simulink model "scars_model."  (R2019b)
settings: Solver=FixedStepAuto  StartTime=0.0  StopTime=TFinal  FixedStep=dT  MaxStep=1  MinStep=dT  RelTol=1e-3
model workspace (MAT data in the model file):
  actuators = 0
values from neighbouring files (symbols this model uses):
  decsec = decyear(2000,1,1,12,0,1) - decyear(2000,1,1,12,0,0)    [SCARSSetup.m]    (also in pwsat2_setup.m; pwsat2_tle.m; scars_setup.m)
  decstart = decyear(utc)    [SCARSSetup.m]    (also in pwsat2_setup.m; pwsat2_tle.m; scars_setup.m)
  forcesBody = [0 0 0]    [SCARSSetup.m]    (also in pwsat2_setup.m; scars_setup.m)
  initMoments = [0 0 0]    [SCARSSetup.m]    (also in pwsat2_setup.m; scars_setup.m)
  momentsBody = [0 0 0]    [SCARSSetup.m]    (also in pwsat2_setup.m; scars_setup.m)
  refEuler = [0 0 1]    [SCARSSetup.m]    (also in pwsat2_setup.m = [0 deg2rad(45) deg2rad(45)]; scars_setup.m)
  refVel = [v_b(1) v_b(2) v_b(3)]    [SCARSSetup.m]    (also in pwsat2_setup.m; scars_setup.m)
  sun_position = getSunPositions(julian, TFinal, dT)    [SCARSSetup.m]    (also in pwsat2_setup.m; scars_setup.m)
  TFinal = 5    [plot_eci2ecef.m]    (also in plot_position.m = 1500; pwsat2_setup.m = 1728000; scars_setup.m = 100)
undefined symbols (not defined in the file or in its folder): gyro, IAU, thruster, WMM2000
libraries: scars_library x12, vrlib x3, simulink x2, simulink_extras x2, aerolibgravity2 x2, aerolibtransform2 x1
settings Model: OrderedModelArguments=off  Creator=asmialek  LastModifiedBy=asmialek
settings DataIOCC: SaveFormat=Array  ReturnWorkspaceOutputsName=scars_out

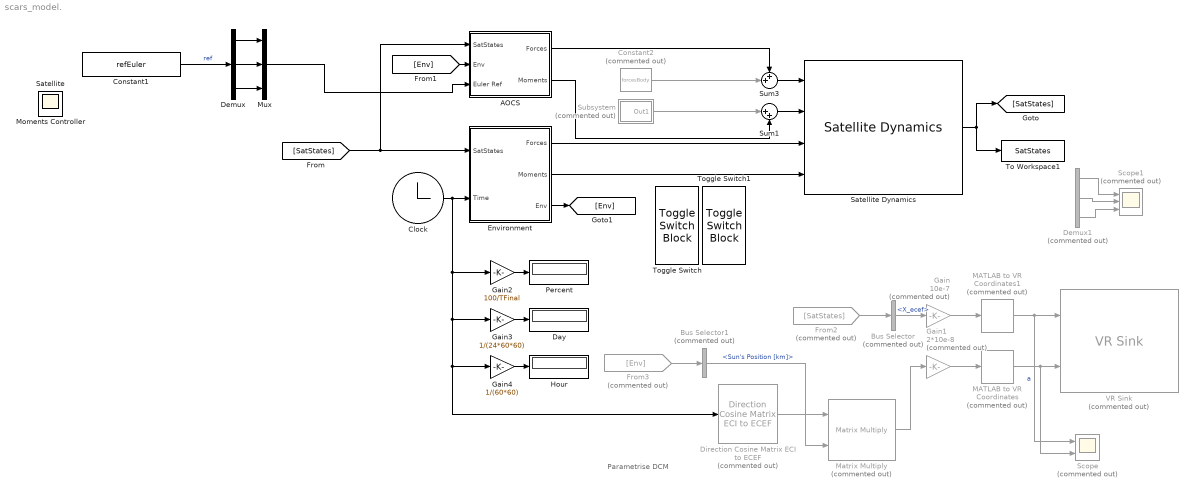
== system scars_model. ==
  note: Parametrise DCM
  AOCS : Subsystem
  Bus Selector : BusSelector  Commented=on  OutputSignals=X_ecef
  Bus Selector1 : BusSelector  Commented=on  OutputSignals=Sun's Position [km]
  Clock : Clock
  Constant1 : Constant  Value=refEuler
  Constant2 : Constant  Commented=on  Value=forcesBody
  Day : Display
  Demux : Demux  Outputs=3
  Demux1 : Demux  Commented=on  Outputs=3
  Direction Cosine Matrix ECI to ECEF : aerolibtransform2/Direction Cosine Matrix ECI to ECEF  Commented=on  red=IAU-2000/2006  year=2000  month=January  day=1  hour=12  min=0  sec=0  deltaT=Sec  errorflag=Error  extraparamflag=off
      settings: AttributesFormatString=%<red>  SourceProductName=Aerospace Blockset  SourceProductBaseCode=AE
  Environment : Subsystem
  From2 : From  Commented=on  GotoTag=SatStates
  From3 : From  Commented=on  GotoTag=Env
  Gain : Gain  Commented=on  Gain=10e-7
  Gain1 : Gain  Commented=on  Gain=2*10e-8
  Gain2 : Gain  Gain=100/TFinal
  Gain3 : Gain  Gain=1/(24*60*60)
  Gain4 : Gain  Gain=1/(60*60)
  Hour : Display
  MATLAB to VR Coordinates : vrlib/Utilities/MATLAB to VR Coordinates  Commented=on
      settings: SourceProductName=Simulink  SourceProductBaseCode=SL
  MATLAB to VR Coordinates1 : vrlib/Utilities/MATLAB to VR Coordinates  Commented=on
      settings: SourceProductName=Simulink  SourceProductBaseCode=SL
  Matrix Multiply : Product  Commented=on  Multiplication=Matrix(*)
  Mux : Mux  Inputs=3
  Percent : Display
  Satellite Dynamics : scars_library/Advanced/Satellite Dynamics  SystemSampleTime=-1  Latency=0  AutoFrameSizeCalculation=off
      link override Moments Switch/Moments: Value=0
  Scope : Scope  Commented=on  NumInputPorts=2
  Scope1 : Scope  Commented=on  NumInputPorts=3
  Subsystem : Subsystem  Commented=on
  Sum1 : Sum  Inputs=|++
  Sum3 : Sum  Inputs=++|
  To Workspace1 : ToWorkspace  VariableName=SatStates  SaveFormat=Timeseries  SampleTime=-1
  Toggle Switch : ToggleSwitchBlock
      settings: Values={{'Off', 'On'}, [0 1]}
  Toggle Switch1 : ToggleSwitchBlock
      settings: Values={{'Off', 'On'}, [0 1]}
  VR Sink : vrlib/VR Sink  Commented=on  InstantiateOnLoad=on  SampleTime=-1  ViewEnable=on  RemoteChange=off  RemoteView=off  FieldsWritten=Sat.translation.3.1.1.double#Sun.translation.3.1.1.double  WorldFileName=sat_test.wrl  AutoView=off  VideoDimensions=[200 320]  AllowVariableSize=off
      settings: SourceProductName=Simulink
  Moments Controller : Scope
  Satellite : Scope
  wires:
  Constant2/1 -> Sum3/2
  Satellite Dynamics/1 -> To Workspace1/1, [SatStates]
  [SatStates] -> AOCS/1(SatStates), Environment/1(SatStates)
  Environment/1(Forces) -> Satellite Dynamics/3
  Environment/2(Moments) -> Satellite Dynamics/4
  Sum3/1 -> Satellite Dynamics/1
  Subsystem/1(Out1) -> Sum1/1
  Sum1/1 -> Satellite Dynamics/2
  Clock/1 -> Direction Cosine Matrix ECI to ECEF/1, Gain4/1, Gain3/1, Gain2/1, Environment/2(Time)
  Environment/3(Env) -> [Env]
  [Env] -> AOCS/2(Env)
  AOCS/1(Forces) -> Sum3/1
  AOCS/2(Moments) -> Sum1/2
  Bus Selector/1 -> Gain/1  "<X_ecef>"
  From2/1 -> Bus Selector/1
  From3/1 -> Bus Selector1/1
  Bus Selector1/1 -> Matrix Multiply/2  "<Sun's Position [km]>"
  MATLAB to VR Coordinates/1 -> Scope/2, VR Sink/2
  MATLAB to VR Coordinates1/1 -> Scope/1, VR Sink/1  "a"
  Gain/1 -> MATLAB to VR Coordinates1/1
  Gain1/1 -> MATLAB to VR Coordinates/1
  Direction Cosine Matrix ECI to ECEF/1 -> Matrix Multiply/1
  Matrix Multiply/1 -> Gain1/1
  Gain2/1 -> Percent/1
  Gain3/1 -> Day/1
  Gain4/1 -> Hour/1
  Constant1/1 -> Demux/1  "ref"
  Demux/2 -> Mux/2
  Demux/3 -> Mux/3
  Demux/1 -> Mux/1
  Mux/1 -> AOCS/3(Euler Ref)
  Demux1/2 -> Scope1/2
  Demux1/1 -> Scope1/1
  Demux1/3 -> Scope1/3

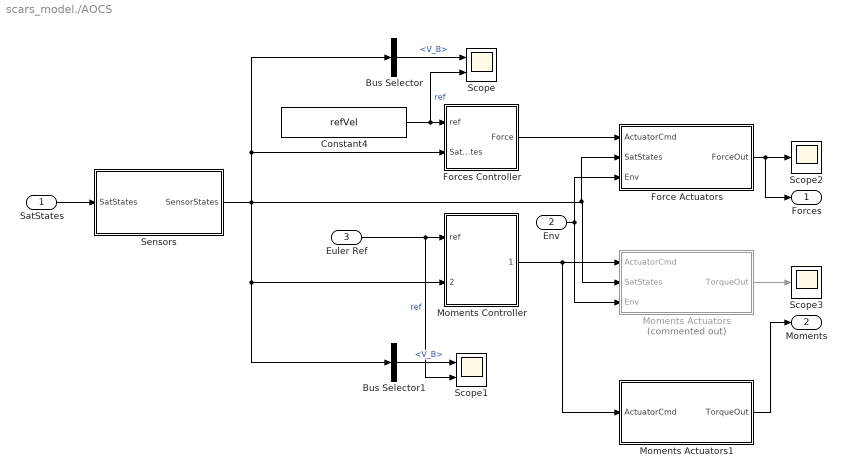
== system scars_model./AOCS ==
  SatStates : Inport
  Env : Inport  Port=2
  Euler Ref : Inport  Port=3
  Bus Selector : BusSelector  OutputSignals=V_B
  Bus Selector1 : BusSelector  OutputSignals=V_B
  Constant4 : Constant  Value=refVel
  Force Actuators : Subsystem
  Forces Controller : Subsystem
  Moments Actuators : Subsystem  Commented=on
  Moments Actuators1 : Subsystem
  Moments Controller : Subsystem
  Scope : Scope  NumInputPorts=2
  Scope1 : Scope  NumInputPorts=2
  Scope2 : Scope
  Scope3 : Scope
  Sensors : Subsystem
  Forces : Outport
  Moments : Outport  Port=2
  wires:
  Force Actuators/1(ForceOut) -> Forces/1, Scope2/1
  SatStates/1 -> Sensors/1(SatStates)
  Constant4/1 -> Scope/2, Forces Controller/1(ref)  "ref"
  Forces Controller/1(Force) -> Force Actuators/1(ActuatorCmd)
  Euler Ref/1 -> Scope1/2, Moments Controller/1(ref)  "ref"
  Bus Selector/1 -> Scope/1  "<V_B>"
  Bus Selector1/1 -> Scope1/1  "<V_B>"
  Moments Actuators/1(TorqueOut) -> Scope3/1
  Sensors/1(SensorStates) -> Bus Selector/1, Forces Controller/2(SatStates), Force Actuators/2(SatStates), Moments Actuators/2(SatStates), Bus Selector1/1, Moments Controller/2(SatStates)
  Env/1 -> Force Actuators/3(Env), Moments Actuators/3(Env)
  Moments Controller/1(Torque) -> Moments Actuators1/1(ActuatorCmd), Moments Actuators/1(ActuatorCmd)
  Moments Actuators1/1(TorqueOut) -> Moments/1

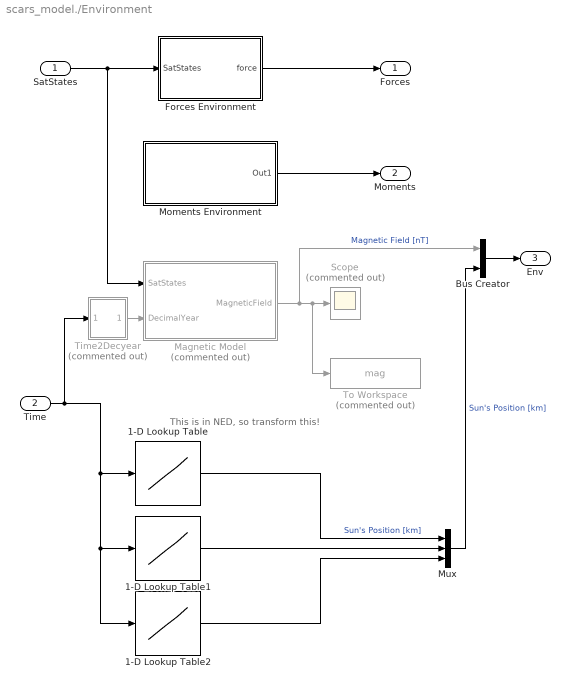
== system scars_model./Environment ==
  note: This is in NED, so transform this!
  SatStates : Inport
  Time : Inport  Port=2
  1-D Lookup Table : Lookup_n-D  NumberOfTableDimensions=1  BreakpointsForDimension1=sun_position(:,1)  Table=sun_position(:,2)  InternalRulePriority=Speed  RndMeth=Simplest  InputSameDT=on
  1-D Lookup Table1 : Lookup_n-D  NumberOfTableDimensions=1  BreakpointsForDimension1=sun_position(:,1)  Table=sun_position(:,3)  InternalRulePriority=Speed  RndMeth=Simplest  InputSameDT=on
  1-D Lookup Table2 : Lookup_n-D  NumberOfTableDimensions=1  BreakpointsForDimension1=sun_position(:,1)  Table=sun_position(:,4)  InternalRulePriority=Speed  RndMeth=Simplest  InputSameDT=on
  Bus Creator : BusCreator  Inputs=2
  Forces Environment : Subsystem
  Magnetic Model : Subsystem  Commented=on
  Moments Environment : Subsystem
  Mux : Mux  Inputs=3
  Scope : Scope  Commented=on
  Time2Decyear : Subsystem  Commented=on
  To Workspace : ToWorkspace  Commented=on  VariableName=mag  SampleTime=-1
  Forces : Outport
  Moments : Outport  Port=2
  Env : Outport  Port=3
  wires:
  SatStates/1 -> Forces Environment/1(SatStates), Magnetic Model/1(SatStates)
  Forces Environment/1(force) -> Forces/1
  Moments Environment/1(Out1) -> Moments/1
  Time2Decyear/1("  ") -> Magnetic Model/2(DecimalYear)
  Magnetic Model/1(MagneticField) -> Bus Creator/1, To Workspace/1, Scope/1  "Magnetic Field [nT]"
  Bus Creator/1 -> Env/1
  1-D Lookup Table2/1 -> Mux/3
  Time/1 -> 1-D Lookup Table2/1, 1-D Lookup Table1/1, 1-D Lookup Table/1, Time2Decyear/1(" ")
  1-D Lookup Table/1 -> Mux/1  "Sun's Position [km]"
  1-D Lookup Table1/1 -> Mux/2
  Mux/1 -> Bus Creator/2  "Sun's Position [km]"

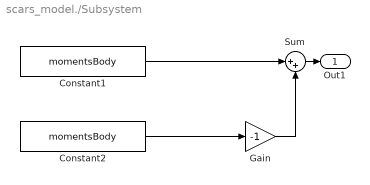
== system scars_model./Subsystem ==
  Constant1 : Constant  Value=momentsBody
  Constant2 : Constant  Value=momentsBody
  Gain : Gain  Gain=-1
  Sum : Sum  Inputs=|++
  Out1 : Outport
  wires:
  Constant1/1 -> Sum/1
  Sum/1 -> Out1/1
  Gain/1 -> Sum/2
  Constant2/1 -> Gain/1

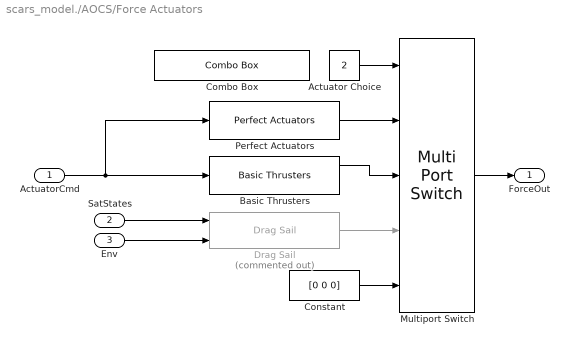
== system scars_model./AOCS/Force Actuators ==
  ActuatorCmd : Inport
  SatStates : Inport  Port=2
  Env : Inport  Port=3
  Actuator Choice : Constant  Value=2
  Basic Thrusters : scars_library/Actuators/Basic Thrusters  SystemSampleTime=-1  Latency=0  AutoFrameSizeCalculation=off
  Combo Box : ComboBox  LabelPosition=Hide  SelectedLabel=Thrusters
      settings: Values={{'Perfect Actuators', 'Thrusters', 'idontknowyet', 'No Actuators'}, [1 2 3 4]}
  Constant : Constant  Value=[0 0 0]
  Drag Sail : scars_library/Actuators/Drag Sail  Commented=on  SystemSampleTime=-1  Latency=0  AutoFrameSizeCalculation=off
  Multiport Switch : MultiPortSwitch  Inputs=4  DiagnosticForDefault=Warning
  Perfect Actuators : scars_library/Actuators/Perfect Actuators  SystemSampleTime=-1  Latency=0  AutoFrameSizeCalculation=off
  ForceOut : Outport
  wires:
  Perfect Actuators/1 -> Multiport Switch/2
  Constant/1 -> Multiport Switch/5
  Actuator Choice/1 -> Multiport Switch/1
  ActuatorCmd/1 -> Perfect Actuators/1, Basic Thrusters/1
  Multiport Switch/1 -> ForceOut/1
  Drag Sail/1 -> Multiport Switch/4
  Basic Thrusters/1 -> Multiport Switch/3
  Env/1 -> Drag Sail/2
  SatStates/1 -> Drag Sail/1

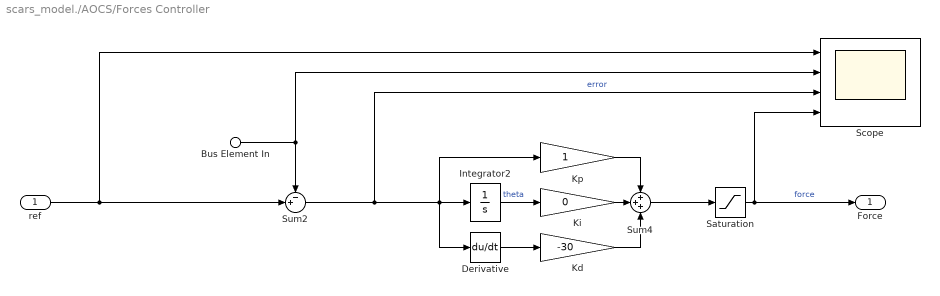
== system scars_model./AOCS/Forces Controller ==
  ref : Inport
  Bus Element In : Inport  Port=2  PortName=SatStates  Element=V_B
  Derivative : Derivative
  Integrator2 : Integrator
  Kd : Gain  Gain=-30
  Ki : Gain  Gain=0
  Kp : Gain
  Saturation : Saturate  UpperLimit=3  LowerLimit=-3
  Scope : Scope  NumInputPorts=4
  Sum2 : Sum  Inputs=-+|
  Sum4 : Sum  Inputs=+++
  Force : Outport
  wires:
  Saturation/1 -> Force/1, Scope/4  "force"
  ref/1 -> Sum2/2, Scope/1
  Sum4/1 -> Saturation/1
  Bus Element In/1 -> Sum2/1, Scope/2
  Kd/1 -> Sum4/3
  Kp/1 -> Sum4/1
  Sum2/1 -> Kp/1, Derivative/1, Integrator2/1, Scope/3  "error"
  Ki/1 -> Sum4/2
  Derivative/1 -> Kd/1
  Integrator2/1 -> Ki/1  "theta"

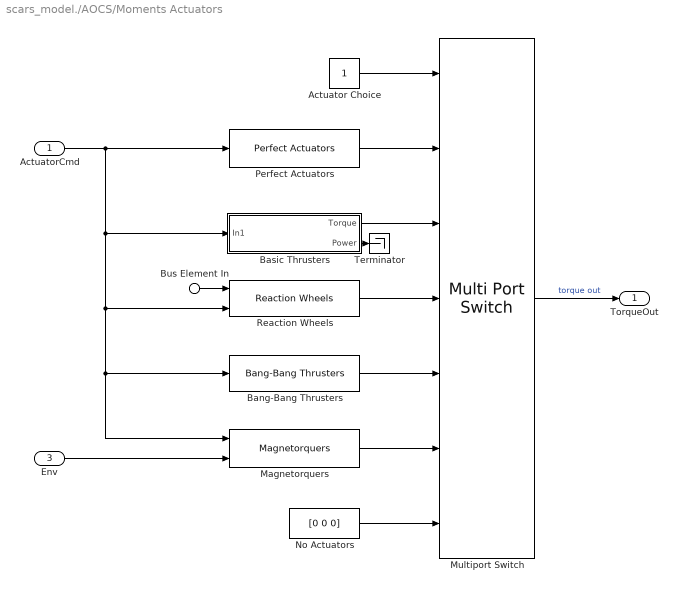
== system scars_model./AOCS/Moments Actuators ==
  ActuatorCmd : Inport
  Bus Element In : Inport  Port=2  PortName=SatStates  Element=V_B
  Env : Inport  Port=3
  Actuator Choice : Constant
  Bang-Bang Thrusters : scars_library/Actuators/Bang-Bang Thrusters  SystemSampleTime=-1  Latency=0  AutoFrameSizeCalculation=off
  Basic Thrusters : Subsystem
  Magnetorquers : scars_library/Actuators/Magnetorquers  SystemSampleTime=-1  Latency=0  AutoFrameSizeCalculation=off
  Multiport Switch : MultiPortSwitch  Inputs=6  DiagnosticForDefault=Warning
  No Actuators : Constant  Value=[0 0 0]
  Perfect Actuators : scars_library/Actuators/Perfect Actuators  SystemSampleTime=-1  Latency=0  AutoFrameSizeCalculation=off
  Reaction Wheels : scars_library/Actuators/Reaction Wheels  SystemSampleTime=-1  Latency=0  AutoFrameSizeCalculation=off
  Terminator : Terminator
  TorqueOut : Outport
  wires:
  Perfect Actuators/1 -> Multiport Switch/2
  Bang-Bang Thrusters/1 -> Multiport Switch/5
  Actuator Choice/1 -> Multiport Switch/1
  Reaction Wheels/1 -> Multiport Switch/4
  Multiport Switch/1 -> TorqueOut/1  "torque out"
  ActuatorCmd/1 -> Perfect Actuators/1, Basic Thrusters/1(In1), Reaction Wheels/2, Magnetorquers/1, Bang-Bang Thrusters/1
  Bus Element In/1 -> Reaction Wheels/1
  Basic Thrusters/1(Torque) -> Multiport Switch/3
  No Actuators/1 -> Multiport Switch/7
  Magnetorquers/1 -> Multiport Switch/6
  Basic Thrusters/2(Power) -> Terminator/1
  Env/1 -> Magnetorquers/2

== system scars_model./AOCS/Moments Actuators1 ==
  ActuatorCmd : Inport
  Perfect Actuators : scars_library/Actuators/Perfect Actuators  SystemSampleTime=-1  Latency=0  AutoFrameSizeCalculation=off
  TorqueOut : Outport
  wires:
  ActuatorCmd/1 -> Perfect Actuators/1
  Perfect Actuators/1 -> TorqueOut/1

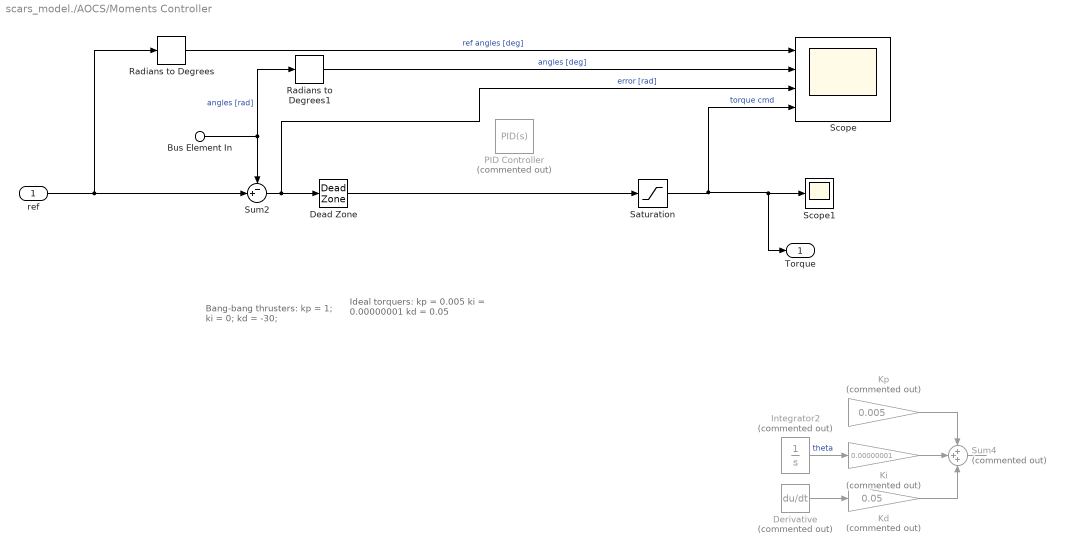
== system scars_model./AOCS/Moments Controller ==
  note: Ideal torquers:
      | kp = 0.005
      | ki = 0.00000001
      | kd = 0.05
  note: Bang-bang thrusters:
      | kp = 1;
      | ki = 0;
      | kd = -30;
  ref : Inport
  Bus Element In : Inport  Port=2  PortName=SatStates  Element=V_B
  Dead Zone : DeadZone  LowerValue=-1e-3  UpperValue=1e-3  SaturateOnIntegerOverflow=on
  Derivative : Derivative  Commented=on
  Integrator2 : Integrator  Commented=on
  Kd : Gain  Commented=on  Gain=0.05
  Ki : Gain  Commented=on  Gain=0.00000001
  Kp : Gain  Commented=on  Gain=0.005
  PID Controller : simulink/Continuous/PID Controller  Commented=on  Controller=PID  Form=Parallel  TimeDomain=Continuous-time  SampleTime=-1  IntegratorMethod=Forward Euler  FilterMethod=Forward Euler  ControllerParametersSource=internal  P=0.005  I=0.00000001  D=0.05  UseFilter=on  N=100  TunerSelectOption=Transfer Function Based (PID Tuner App)  InitialConditionSource=internal  InitialConditionForIntegrator=0  InitialConditionForFilter=0  DifferentiatorICPrevScaledInput=0  ExternalReset=none  TrackingMode=off  Kt=1  LimitOutput=off  UpperSaturationLimit=inf  LowerSaturationLimit=-inf  LinearizeAsGain=on  AntiWindupMode=none  Kb=1  POutMin=[]  POutMax=[]  IOutMin=[]  IOutMax=[]  DOutMin=[]  DOutMax=[]  NOutMin=[]  NOutMax=[]  SumOutMin=[]  SumOutMax=[]  SaturationOutMin=[]  SaturationOutMax=[]  PParamMin=[]  PParamMax=[]  IParamMin=[]  IParamMax=[]  DParamMin=[]  DParamMax=[]  NParamMin=[]  NParamMax=[]  KbParamMin=[]  KbParamMax=[]  KtParamMin=[]  KtParamMax=[]  KbOutMin=[]  KbOutMax=[]  KtOutMin=[]  KtOutMax=[]  IntegratorOutMin=[]  IntegratorOutMax=[]  FilterOutMin=[]  FilterOutMax=[]  SumI1OutMin=[]  SumI1OutMax=[]  SumI2OutMin=[]  SumI2OutMax=[]  SumI3OutMin=[]  SumI3OutMax=[]  SumI4OutMin=[]  SumI4OutMax=[]  SumDOutMin=[]  SumDOutMax=[]  DifferentiatorOutMin=[]  DifferentiatorOutMax=[]  FilterDiffOutCoefMin=[]  FilterDiffOutCoefMax=[]  ReciprocalOutMin=[]  ReciprocalOutMax=[]  SumDenOutMin=[]  SumDenOutMax=[]  SumNumOutMin=[]  SumNumOutMax=[]  DivideOutMin=[]  DivideOutMax=[]  IntegratorContinuousStateAttributes=''  IntegratorStateMustResolveToSignalObject=off  IntegratorRTWStateStorageClass=Auto  FilterContinuousStateAttributes=''  FilterStateMustResolveToSignalObject=off  FilterRTWStateStorageClass=Auto  ParallelPVariant=InternalParameters  IdealPVariant=Disabled  IVariant=InternalParameters  DVariant=InternalParameters  IntegratorVariant=Continuous  SatVariant=Disabled  AWVariant=Passthrough  PCopyVariant=Disabled  TRVariant=Disabled  FdbkBlocksVariant=Forward  IdealPFdbkVariant=Disabled  SatFdbkVariant=Disabled  DerivativeFilterVariant=ContFilter  NVariant=InternalParameters  NCopyVariant=Disabled  FilterICVariant=InternalICsFilter  IntegratorICVariant=InternalICs  ExternalResetVariant=Disabled  TRSumVariant=Passthrough  SumFdbkVariant=Disabled  SumVariant=Sum_PID
  Radians to Degrees : simulink_extras/Transformations/Radians to Degrees
  Radians to Degrees1 : simulink_extras/Transformations/Radians to Degrees
  Saturation : Saturate  UpperLimit=3  LowerLimit=-3
  Scope : Scope  NumInputPorts=4
  Scope1 : Scope
  Sum2 : Sum  Inputs=-+|
  Sum4 : Sum  Commented=on  Inputs=+++
  Torque : Outport
  wires:
  Saturation/1 -> Torque/1, Scope1/1, Scope/4  "torque cmd"
  ref/1 -> Sum2/2, Radians to Degrees/1
  Bus Element In/1 -> Sum2/1, Radians to Degrees1/1  "angles [rad]"
  Radians to Degrees/1 -> Scope/1  "ref angles [deg]"
  Radians to Degrees1/1 -> Scope/2  "angles [deg]"
  Sum2/1 -> Scope/3, Dead Zone/1  "error [rad]"
  Ki/1 -> Sum4/2
  ? -> Kp/1, Derivative/1, Integrator2/1
  Sum4/1 -> ?
  Kp/1 -> Sum4/1
  Kd/1 -> Sum4/3
  Integrator2/1 -> Ki/1  "theta"
  Derivative/1 -> Kd/1
  Dead Zone/1 -> Saturation/1

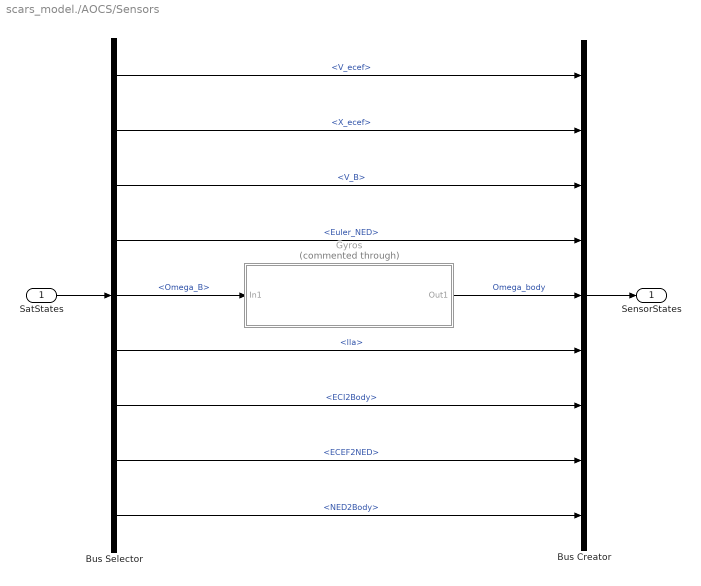
== system scars_model./AOCS/Sensors ==
  SatStates : Inport
  Bus Creator : BusCreator  Inputs=9
  Bus Selector : BusSelector  OutputSignals=V_ecef,X_ecef,V_B,Euler_NED,Omega_B,lla,ECI2Body,ECEF2NED,NED2Body
  Gyros : Subsystem  Commented=through
  SensorStates : Outport
  wires:
  SatStates/1 -> Bus Selector/1
  Bus Creator/1 -> SensorStates/1
  Bus Selector/7 -> Bus Creator/7  "<ECI2Body>"
  Bus Selector/8 -> Bus Creator/8  "<ECEF2NED>"
  Bus Selector/9 -> Bus Creator/9  "<NED2Body>"
  Bus Selector/6 -> Bus Creator/6  "<lla>"
  Bus Selector/5 -> Gyros/1(In1)  "<Omega_B>"
  Bus Selector/1 -> Bus Creator/1  "<V_ecef>"
  Gyros/1(Out1) -> Bus Creator/5  "Omega_body"
  Bus Selector/2 -> Bus Creator/2  "<X_ecef>"
  Bus Selector/3 -> Bus Creator/3  "<V_B>"
  Bus Selector/4 -> Bus Creator/4  "<Euler_NED>"

== system scars_model./Environment/Forces Environment ==
  SatStates : Inport
  Subsystem : Subsystem
  force : Outport
  wires:
  Subsystem/1(Out1) -> force/1
  SatStates/1 -> Subsystem/1(SatStates)

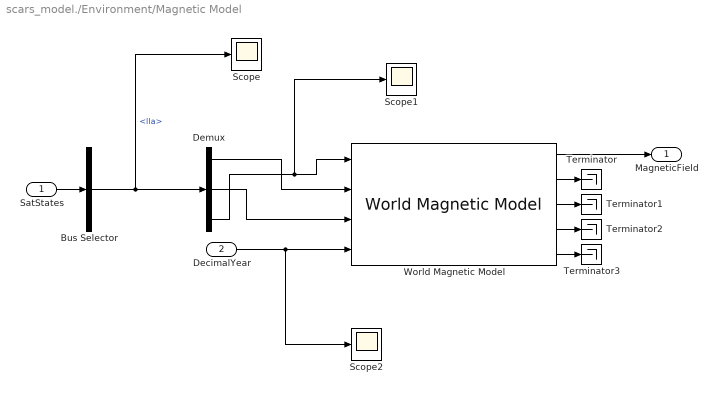
== system scars_model./Environment/Magnetic Model ==
  SatStates : Inport
  DecimalYear : Inport  Port=2
  Bus Selector : BusSelector  OutputSignals=lla
  Demux : Demux  Outputs=3
  Scope : Scope
  Scope1 : Scope
  Scope2 : Scope
  Terminator{,1..3} (4 alike) : Terminator
  World Magnetic Model : aerolibgravity2/World Magnetic Model  model=WMM2000 (2000-2005)  customFile='WMM2015v2.COF'  units=Metric (MKS)  time_in=on  month=January  day=1  year=2015  action=Error  h_out=on  dec_out=on  inc_out=on  ti_out=on
      settings: SourceProductName=Aerospace Blockset  SourceProductBaseCode=AE
  MagneticField : Outport
  wires:
  SatStates/1 -> Bus Selector/1
  DecimalYear/1 -> Scope2/1, World Magnetic Model/4
  World Magnetic Model/1 -> MagneticField/1
  World Magnetic Model/2 -> Terminator/1
  World Magnetic Model/5 -> Terminator3/1
  World Magnetic Model/3 -> Terminator1/1
  World Magnetic Model/4 -> Terminator2/1
  Bus Selector/1 -> Demux/1, Scope/1  "<lla>"
  Demux/1 -> World Magnetic Model/2
  Demux/2 -> World Magnetic Model/3
  Demux/3 -> Scope1/1, World Magnetic Model/1

== system scars_model./Environment/Moments Environment ==
  Constant : Constant  Value=initMoments
  Out1 : Outport
  wires:
  Constant/1 -> Out1/1

== system scars_model./Environment/Time2Decyear ==
  " " : Inport
  Decsec : Gain  Gain=decsec
  Initial Decyear : Constant  Value=decstart
  Sum : Sum  Inputs=|++
  "  " : Outport
  wires:
  Initial Decyear/1 -> Sum/1
  " "/1 -> Decsec/1
  Decsec/1 -> Sum/2
  Sum/1 -> "  "/1

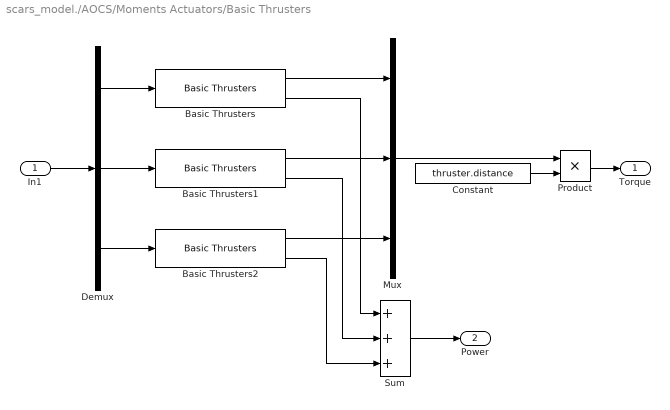
== system scars_model./AOCS/Moments Actuators/Basic Thrusters ==
  In1 : Inport
  Basic Thrusters : scars_library/Actuators/Basic Thrusters  SystemSampleTime=-1  Latency=0  AutoFrameSizeCalculation=off
  Basic Thrusters1 : scars_library/Actuators/Basic Thrusters  SystemSampleTime=-1  Latency=0  AutoFrameSizeCalculation=off
  Basic Thrusters2 : scars_library/Actuators/Basic Thrusters  SystemSampleTime=-1  Latency=0  AutoFrameSizeCalculation=off
  Constant : Constant  Value=thruster.distance
  Demux : Demux  Outputs=3
  Mux : Mux  Inputs=3
  Product : Product
  Sum : Sum  Inputs=+++
  Torque : Outport
  Power : Outport  Port=2
  wires:
  In1/1 -> Demux/1
  Demux/1 -> Basic Thrusters/1
  Basic Thrusters/1 -> Mux/1
  Basic Thrusters1/1 -> Mux/2
  Basic Thrusters2/1 -> Mux/3
  Basic Thrusters/2 -> Sum/1
  Basic Thrusters2/2 -> Sum/3
  Basic Thrusters1/2 -> Sum/2
  Constant/1 -> Product/2
  Mux/1 -> Product/1
  Product/1 -> Torque/1
  Sum/1 -> Power/1
  Demux/2 -> Basic Thrusters1/1
  Demux/3 -> Basic Thrusters2/1

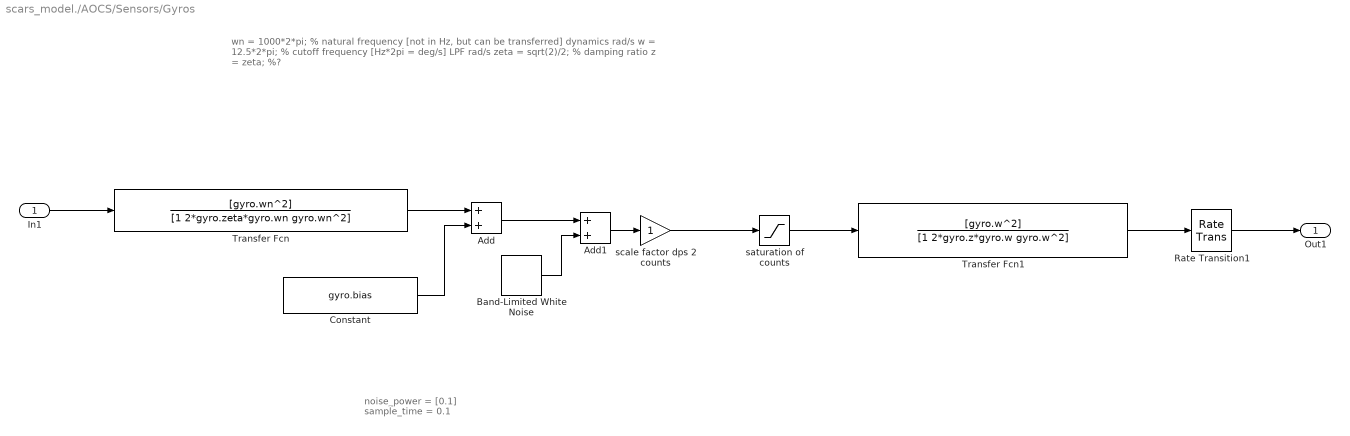
== system scars_model./AOCS/Sensors/Gyros ==
  note: noise_power  = [0.1]
      | sample_time = 0.1
  note: wn = 1000*2*pi; % natural frequency [not in Hz, but can be transferred] dynamics rad/s
      | w = 12.5*2*pi; % cutoff frequency [Hz*2pi = deg/s] LPF rad/s
      | zeta = sqrt(2)/2; % damping ratio
      | z = zeta; %?
  In1 : Inport
  Add : Sum
  Add1 : Sum
  Band-Limited White Noise : simulink/Sources/Band-Limited White Noise  Cov=[gyro.noise_power]  Ts=gyro.sample_time  seed=[23341]
  Constant : Constant  Value=gyro.bias
  Rate Transition1 : RateTransition  OutPortSampleTime=gyro.rate
  Transfer Fcn : TransferFcn  Numerator=[gyro.wn^2]  Denominator=[1 2*gyro.zeta*gyro.wn gyro.wn^2]
  Transfer Fcn1 : TransferFcn  Numerator=[gyro.w^2]  Denominator=[1 2*gyro.z*gyro.w gyro.w^2]
  saturation of counts : Saturate  UpperLimit=gyro.max  LowerLimit=gyro.min
  scale factor dps 2 counts : Gain
  Out1 : Outport
  wires:
  Transfer Fcn/1 -> Add/1
  Constant/1 -> Add/2
  Add/1 -> Add1/1
  Band-Limited White Noise/1 -> Add1/2
  Add1/1 -> scale factor dps 2 counts/1
  scale factor dps 2 counts/1 -> saturation of counts/1
  saturation of counts/1 -> Transfer Fcn1/1
  Transfer Fcn1/1 -> Rate Transition1/1
  In1/1 -> Transfer Fcn/1
  Rate Transition1/1 -> Out1/1

== system scars_model./Environment/Forces Environment/Subsystem ==
  Bus Element In : Inport  PortName=SatStates  Element=X_ecef
  Spherical Harmonic Gravity Model1 : aerolibgravity2/Spherical Harmonic Gravity Model  units=Metric (MKS)  degree=120  action=Warning  ptype=EGM2008  datafile='aerogmm2b.mat'
      settings: SourceProductName=Aerospace Blockset  SourceProductBaseCode=AE
  To Workspace13 : ToWorkspace  VariableName=g  SampleTime=-1
  Out1 : Outport
  wires:
  Bus Element In/1 -> Spherical Harmonic Gravity Model1/1
  Spherical Harmonic Gravity Model1/1 -> Out1/1, To Workspace13/1
